simulink model "Clase2"  (Simulink 7.2)
settings: Solver=ode45  StartTime=0.0  StopTime=100.0  RelTol=1e-3
values from neighbouring files (symbols this model uses):
  A1 = 20    [GlobalParam.m]    (also in GlobalParam2.m = 10)
  A2 = 30    [GlobalParam.m]    (also in GlobalParam2.m = 12)
  R1 = 15    [GlobalParam.m]    (also in GlobalParam2.m)
  R2 = 25    [GlobalParam.m]    (also in GlobalParam2.m = 15)
settings Model: Creator=ALan  LastModifiedBy=ALan

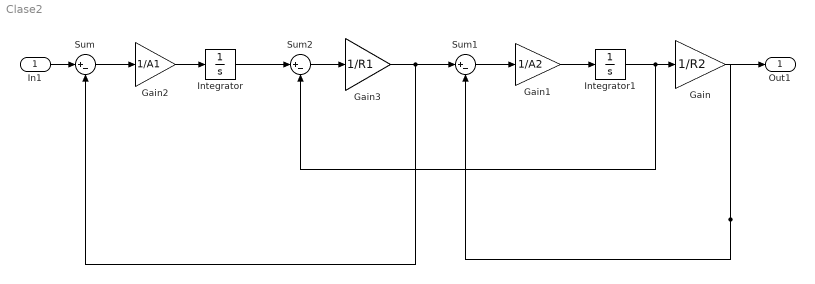
== system Clase2 ==
  In1 : Inport  OutDataType=sfix(16)  OutScaling=2^0
  Gain : Gain  Gain=1/R2  ParameterDataType=sfix(16)  ParameterScaling=2^0  OutDataType=sfix(16)  OutScaling=2^0
  Gain1 : Gain  Gain=1/A2  ParameterDataType=sfix(16)  ParameterScaling=2^0  OutDataType=sfix(16)  OutScaling=2^0
  Gain2 : Gain  Gain=1/A1  ParameterDataType=sfix(16)  ParameterScaling=2^0  OutDataType=sfix(16)  OutScaling=2^0
  Gain3 : Gain  Gain=1/R1  ParameterDataType=sfix(16)  ParameterScaling=2^0  OutDataType=sfix(16)  OutScaling=2^0
  Integrator : Integrator
  Integrator1 : Integrator
  Sum : Sum  Inputs=|+-  OutDataType=sfix(16)  OutScaling=2^0
  Sum1 : Sum  Inputs=|+-  OutDataType=sfix(16)  OutScaling=2^0
  Sum2 : Sum  Inputs=|+-  OutDataType=sfix(16)  OutScaling=2^0
  Out1 : Outport  OutDataType=sfix(16)  OutScaling=2^0
  wires:
  Gain2/1 -> Integrator/1
  Sum/1 -> Gain2/1
  Integrator/1 -> Sum2/1
  Sum2/1 -> Gain3/1
  Gain3/1 -> Sum1/1, Sum/2
  Sum1/1 -> Gain1/1
  Gain1/1 -> Integrator1/1
  Integrator1/1 -> Gain/1, Sum2/2
  Gain/1 -> Out1/1, Sum1/2
  In1/1 -> Sum/1
